simulink model "LQSwingup"  (R2019b)
settings: Solver=ode1  StartTime=0.0  StopTime=inf  FixedStep=0.002  RelTol=1e-3  EnableMultiTasking=on
PostLoadFcn:
  | qc_set_target_type(getConfigSet(bdroot, 'QUARC Default Target Configuration'));
undefined symbols (not defined in the file): HIL, Klqi_int, Klqi_state, Parameters, qc_get_step_size
libraries: quarc_library x4
settings Model: SimulationMode=external  ExtModeTrigDuration=5000  Creator=CFulford  LastModifiedBy=Student
settings SolverCC: PositivePriorityOrder=on
settings DataIOCC: LimitDataPoints=on  SaveFormat=Array  SignalLoggingSaveFormat=ModelDataLogs  ReturnWorkspaceOutputs=off
settings OptimizationCC: ExpressionDepthLimit=2147483647  InitFltsAndDblsToZero=on  LifeSpan=inf
settings DebuggingCC: SaveWithParameterizedLinksMsg=none  UnderspecifiedInitializationDetection=Classic  MergeDetectMultiDrivingBlocksExec=none  SolverPrmCheckMsg=warning  MultiTaskDSMMsg=warning  MultiTaskCondExecSysMsg=none  FcnCallInpInsideContextMsg=warning  StateNameClashWarn=warning  SFUnexpectedBacktrackingDiag=warning  SFNoUnconditionalDefaultTransitionDiag=warning  SFExecutionAtInitializationDiag=none  ArithmeticOperatorsInVariantConditions=warning
settings HardwareCC: ProdBitPerPointer=32  ProdBitPerSizeT=32  ProdBitPerPtrDiffT=32  ProdLargestAtomicFloat=None  ProdIntDivRoundTo=Undefined  ProdEndianess=Unspecified  ProdWordSize=32  ProdHWDeviceType=32-bit Generic
settings ModelReferenceCC: PropagateSignalLabelsOutOfModel=off
settings SFSimCC: SimUseLocalCustomCode=off  CustomCodeUndefinedFunction=UseInterfaceOnly
settings RTWCC: Description=QUARC Win64 Target  SystemTargetFile=quarc_win64.tlc  TemplateMakefile=quarc_default_tmf  RTWUseLocalCustomCode=off
settings CodeAppCC: StateflowObjectComments=on
settings STFCustomTargetCC: TargetPreCompLibLocation=C:\PROGRA~3\QUARC\lib\2019b\win64\release  ConcurrentExecutionCompliant=on  GeneratePreprocessorConditionals=Disable all  CombineOutputUpdateFcns=on  CPPClassGenCompliant=on  SystemTargetFile=quarc_win64.tlc
settings GRTTargetCC: TargetPreCompLibLocation=C:\PROGRA~3\QUARC\lib\2019b\win64\release  TargetLangStandard=C89/C90 (ANSI)  ParMdlRefBuildCompliant=off  CompOptLevelCompliant=off  GeneratePreprocessorConditionals=Disable all  MatFileLogging=off  UseToolchainInfoCompliant=off  ExtMode=on  ExtModeMexFile=quarc_comm
settings ConfigComp: CovMetricSettings=dw  CovHtmlReporting=on  CovSaveCumulativeToWorkspaceVar=on  CovSaveSingleToWorkspaceVar=on  CovExternalEMLEnable=off  CovSFcnEnable=off

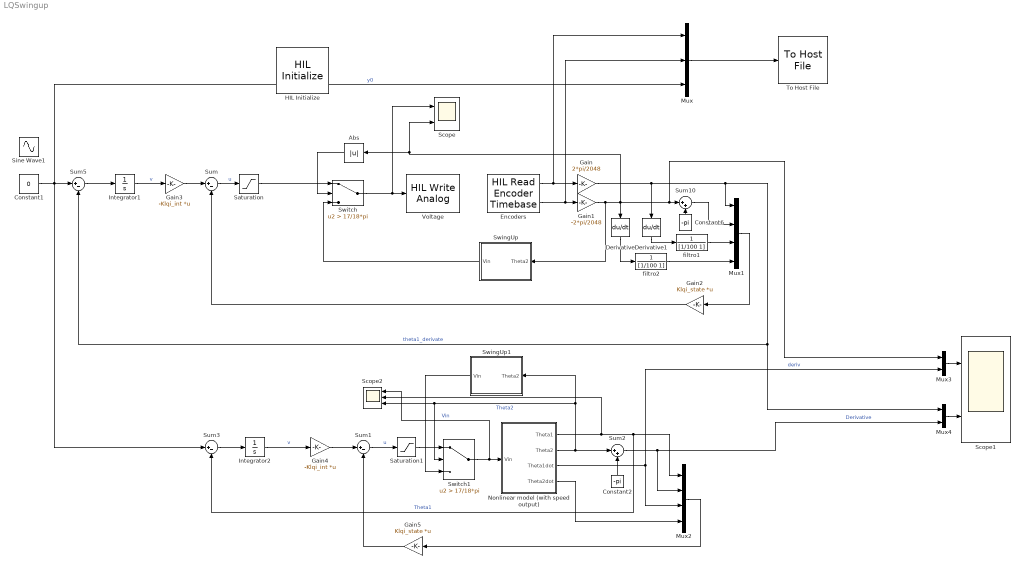
== system LQSwingup ==
  Abs : Abs
  Constant1 : Constant  Value=0
  Constant2 : Constant  Value=-pi
  Constant6 : Constant  Value=-pi
  Derivative : Derivative
  Derivative1 : Derivative
  Encoders : quarc_library/Data Acquisition/Generic/Timebases/HIL Read Encoder Timebase  object_name=HIL-1  clock=0  channels=[0:1]  samples_in_buffer=max(ceil(1/qc_get_step_size), 1)  active=on  vector_output=off  data_type_mode=Inherit via back propagation  data_type=double
  Gain : Gain  Gain=2*pi/2048
  Gain1 : Gain  Gain=-2*pi/2048
  Gain2 : Gain  Gain=Klqi_state  Multiplication=Matrix(K*u)
  Gain3 : Gain  Gain=-Klqi_int  Multiplication=Matrix(K*u)
  Gain4 : Gain  Gain=-Klqi_int  Multiplication=Matrix(K*u)
  Gain5 : Gain  Gain=Klqi_state  Multiplication=Matrix(K*u)
  HIL Initialize : quarc_library/Data Acquisition/Generic/Configuration/HIL Initialize  Priority=-99  object_name=HIL-1  board_type=qube_servo2_usb  board_number=0  board_options=""  exclusive=off  active=off  hardware_clocks=[0]  clock_modes=[]  initial_clock_frequencies=[]  set_clock_params_at_start=off  set_clock_params_at_switch_in=off  set_clock_frequencies_at_start=off  set_clock_frequencies_at_switch_in=off  analog_input_channels=[0]  analog_input_configurations=[]  analog_input_maximums=3  analog_input_minimums=-3  set_analog_input_params_at_start=off  set_analog_input_params_at_switch_in=off  analog_output_channels=[0]  analog_output_maximums=15  analog_output_minimums=-15  initial_analog_outputs=[0]  final_analog_outputs=[0]  watchdog_analog_outputs=0  set_analog_output_params_at_start=off  set_analog_output_params_at_switch_in=off  set_analog_outputs_at_start=on  set_analog_outputs_at_switch_in=off  set_analog_outputs_at_terminate=on  set_analog_outputs_at_switch_out=off  set_analog_outputs_on_watchdog=on  digital_input_channels=[]  digital_output_channels=[0]  digital_output_configuration=[]  initial_digital_outputs=[1]  final_digital_outputs=[0]  watchdog_digital_outputs=[0]  set_digital_output_params_at_start=off  set_digital_output_params_at_switch_in=off  set_digital_outputs_at_start=on  set_digital_outputs_at_switch_in=off  set_digital_outputs_at_terminate=on  set_digital_outputs_at_switch_out=off  set_digital_outputs_on_watchdog=on  encoder_channels=[0:1]  quadrature=[4]  encoder_filter_frequency=[]  initial_encoder_counts=[0]  set_encoder_params_at_start=off  set_encoder_params_at_switch_in=off  set_encoder_counts_at_start=on  set_encoder_counts_at_switch_in=off  pwm_channels=[]  pwm_modes=[]  pwm_frequency=[]  pwm_configuration=[]  pwm_alignment=[]  pwm_polarity=[]  pwm_leading_deadband=[]  pwm_trailing_deadband=[]  initial_pwm_outputs=[]  final_pwm_outputs=[]  watchdog_pwm_outputs=[]  set_pwm_params_at_start=off  set_pwm_params_at_switch_in=off  set_pwm_outputs_at_start=off  set_pwm_outputs_at_switch_in=off  set_pwm_outputs_at_terminate=off  set_pwm_outputs_at_switch_out=off  set_pwm_outputs_on_watchdog=off  other_output_channels=[11000:11002]  initial_other_outputs=[0 1 0]  final_other_outputs=[1 0 0]  watchdog_other_outputs=[0 0 1]  set_other_outputs_at_start=on  set_other_outputs_at_switch_in=off  set_other_outputs_at_terminate=on  set_other_outputs_at_switch_out=off  set_other_outputs_on_watchdog=on
  Integrator1 : Integrator
  Integrator2 : Integrator
  Mux : Mux  Inputs=3
  Mux1 : Mux
  Mux2 : Mux
  Mux3 : Mux  Inputs=2
  Mux4 : Mux  Inputs=2
  Nonlinear model (with speed output) : Subsystem
  Saturation : Saturate  UpperLimit=10  LowerLimit=-10
  Saturation1 : Saturate  UpperLimit=10  LowerLimit=-10
  Scope : Scope  NumInputPorts=2
  Scope1 : Scope  NumInputPorts=2
  Scope2 : Scope  NumInputPorts=3
  Sine Wave1 : Sin  SampleTime=0
  Sum{,1,3,5} (4 alike) : Sum  Inputs=|+-
  Sum10 : Sum  Inputs=|++
  Sum2 : Sum  Inputs=|++
  SwingUp : Subsystem
  SwingUp1 : Subsystem
  Switch : Switch  Criteria=u2 > Threshold  Threshold=17/18*pi
  Switch1 : Switch  Criteria=u2 > Threshold  Threshold=17/18*pi
  To Host File : quarc_library/Sinks/To Host/To Host File  file_name=data_%{date}_%{time}.mat  variable_name=data_%{date}_%{time}  decimation=1  sample_time=-1  file_format=MAT-file v.5  options=No header or footer  append=off  final_file_name=data_17-May-2024_12-50-43.mat  bitrate=2000000
  Voltage : quarc_library/Data Acquisition/Generic/Immediate I//O/HIL Write Analog  object_name=HIL-1  channels=0  sample_time=-1  active=off  vector_input=off
  "filtro1 " : TransferFcn  Denominator=[1/100 1]
  filtro2 : TransferFcn  Denominator=[1/100 1]
  wires:
  Mux/1 -> To Host File/1
  Gain2/1 -> Sum/2
  Encoders/2 -> Mux/2, Gain1/1
  Switch/1 -> Scope/1, Voltage/1
  Mux1/1 -> Gain2/1
  Mux3/1 -> Scope1/1
  "filtro1 "/1 -> Mux1/3
  Sum10/1 -> Mux1/2
  Gain3/1 -> Sum/1
  Derivative/1 -> filtro2/1
  Mux4/1 -> Scope1/2
  Derivative1/1 -> "filtro1 "/1
  Encoders/1 -> Mux/1, Gain/1
  Sum/1 -> Saturation/1  "u"
  Integrator1/1 -> Gain3/1  "v"
  filtro2/1 -> Mux1/4
  Gain/1 -> Sum5/2, Mux4/1, Mux1/1, Derivative1/1  "theta1_derivate"
  Sum5/1 -> Integrator1/1
  Constant6/1 -> Sum10/2
  Saturation/1 -> Switch/1
  Gain1/1 -> SwingUp/1(Theta2), Scope/2, Abs/1, Mux3/1, Sum10/1, Derivative/1
  SwingUp/1(Vin) -> Switch/3
  Nonlinear model (with speed output)/1(Theta1) -> Scope2/2, Mux2/1, Sum3/2  "Theta1"
  Saturation1/1 -> Switch1/1
  SwingUp1/1(Vin) -> Switch1/3
  Sum1/1 -> Saturation1/1  "u"
  Switch1/1 -> Scope2/1, Nonlinear model (with speed output)/1(Vin)  "Vin"
  Constant1/1 -> Mux/3, Sum3/1, Sum5/1  "y0"
  Nonlinear model (with speed output)/2(Theta2) -> Sum2/1, SwingUp1/1(Theta2), Switch1/2, Scope2/3  "Theta2"
  Nonlinear model (with speed output)/4(Theta2dot) -> Mux2/4
  Constant2/1 -> Sum2/2
  Nonlinear model (with speed output)/3(Theta1dot) -> Mux3/2, Mux2/3  "deriv"
  Sum3/1 -> Integrator2/1
  Sum2/1 -> Mux4/2, Mux2/2  "Derivative"
  Gain5/1 -> Sum1/2
  Integrator2/1 -> Gain4/1  "v"
  Mux2/1 -> Gain5/1
  Gain4/1 -> Sum1/1
  Abs/1 -> Switch/2

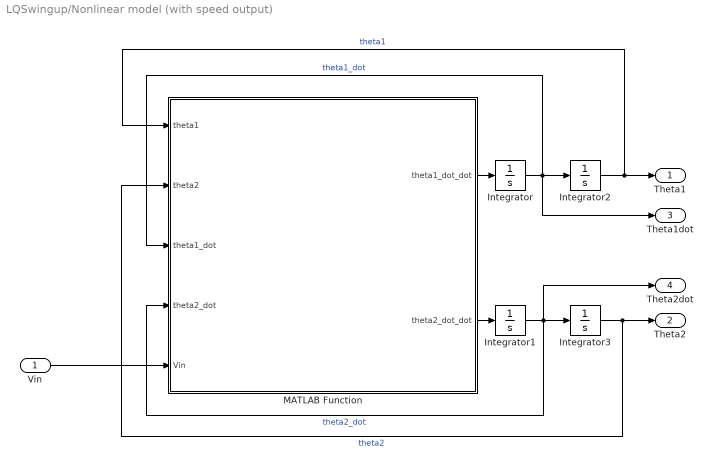
== system LQSwingup/Nonlinear model (with speed output) ==
  Vin : Inport
  Integrator{,1..3} (4 alike) : Integrator
  MATLAB Function : MATLAB Function  TreatAsAtomicUnit=on  mask{Pars=Parameters}
      mask prompts: Pars "Struct containing model parameters"
  Theta1 : Outport
  Theta2 : Outport  Port=2
  Theta1dot : Outport  Port=3
  Theta2dot : Outport  Port=4
  wires:
  Integrator/1 -> Theta1dot/1, MATLAB Function/3(theta1_dot), Integrator2/1  "theta1_dot"
  Integrator1/1 -> Theta2dot/1, MATLAB Function/4(theta2_dot), Integrator3/1  "theta2_dot"
  MATLAB Function/1(theta1_dot_dot) -> Integrator/1
  Integrator3/1 -> Theta2/1, MATLAB Function/2(theta2)  "theta2"
  MATLAB Function/2(theta2_dot_dot) -> Integrator1/1
  Integrator2/1 -> MATLAB Function/1(theta1), Theta1/1  "theta1"
  Vin/1 -> MATLAB Function/5(Vin)

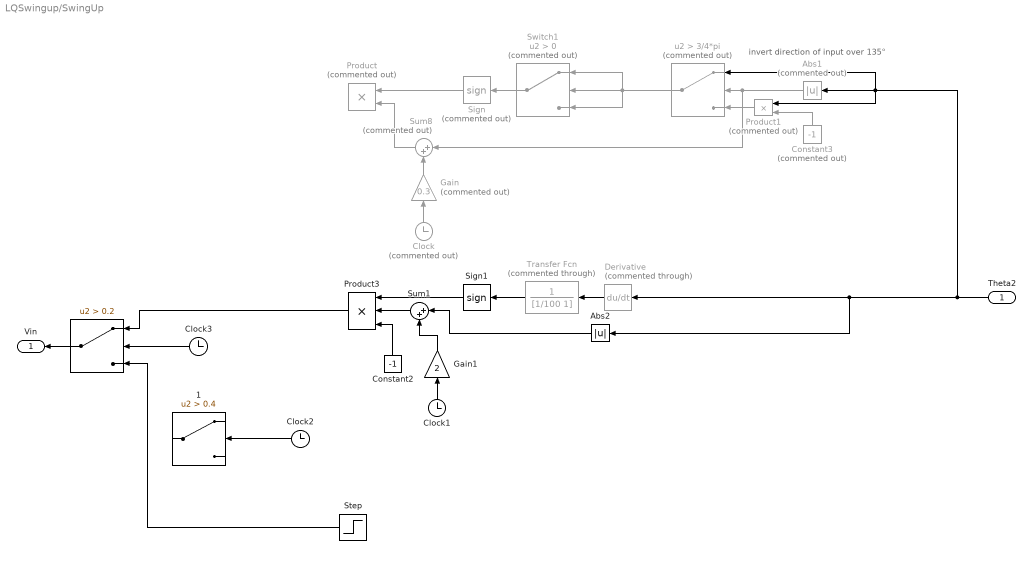
== system LQSwingup/SwingUp ==
  note: invert direction of input over 135°
  Theta2 : Inport
  " " : Switch  Commented=on  Criteria=u2 > Threshold  Threshold=3/4*pi
  " " : Switch  Criteria=u2 > Threshold  Threshold=0.2
  " 1" : Switch  Criteria=u2 > Threshold  Threshold=0.4
  Abs1 : Abs  Commented=on
  Abs2 : Abs
  Clock : Clock  Commented=on
  Clock1 : Clock
  Clock2 : Clock
  Clock3 : Clock
  Constant2 : Constant  Value=-1
  Constant3 : Constant  Commented=on  Value=-1
  Derivative : Derivative  Commented=through
  Gain : Gain  Commented=on  Gain=0.3
  Gain1 : Gain  Gain=2
  Product : Product  Commented=on
  Product1 : Product  Commented=on
  Product3 : Product  Inputs=3
  Sign : Signum  Commented=on
  Sign1 : Signum
  Step : Step  Time=0  SampleTime=0
  Sum1 : Sum  Inputs=|++
  Sum8 : Sum  Commented=on  Inputs=|++
  Switch1 : Switch  Commented=on  Criteria=u2 > Threshold
  Transfer Fcn : TransferFcn  Commented=through  Denominator=[1/100 1]
  Vin : Outport
  wires:
  Abs1/1 -> Sum8/1, " "/2
  " "/1 -> Switch1/3, Switch1/2, Switch1/1
  Constant3/1 -> Product1/2
  Clock/1 -> Gain/1
  Product1/1 -> " "/3
  Switch1/1 -> Sign/1
  Gain/1 -> Sum8/2
  Sign/1 -> Product/1
  Sum8/1 -> Product/2
  Sign1/1 -> Product3/1
  Sum1/1 -> Product3/2
  Clock1/1 -> Gain1/1
  Gain1/1 -> Sum1/2
  Constant2/1 -> Product3/3
  " "/1 -> Vin/1
  Product3/1 -> " "/1
  Clock2/1 -> " 1"/2
  Clock3/1 -> " "/2
  Abs2/1 -> Sum1/1
  Theta2/1 -> Product1/1, Abs1/1, " "/1, Derivative/1, Abs2/1
  Derivative/1 -> Transfer Fcn/1
  Transfer Fcn/1 -> Sign1/1
  Step/1 -> " "/3

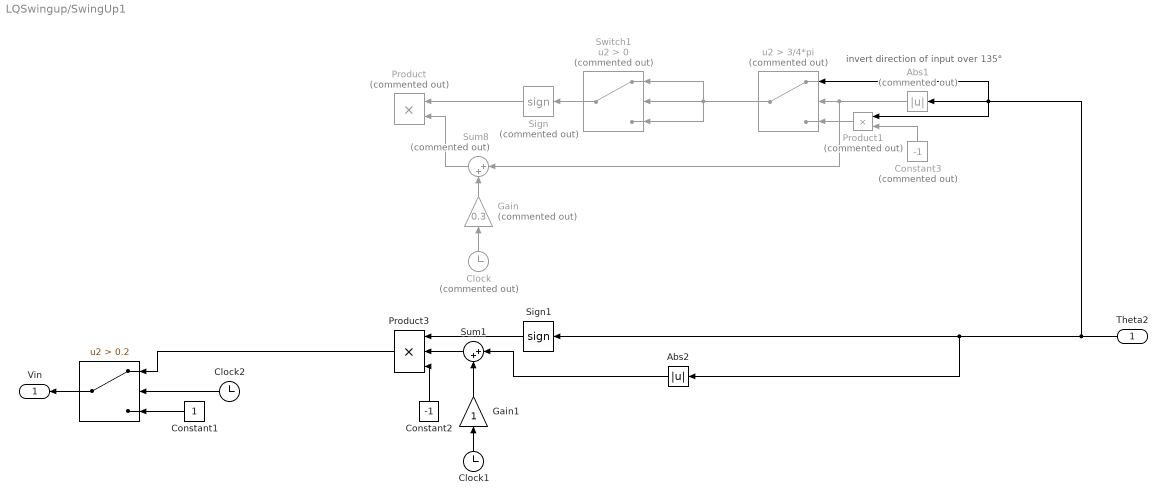
== system LQSwingup/SwingUp1 ==
  note: invert direction of input over 135°
  Theta2 : Inport
  " " : Switch  Commented=on  Criteria=u2 > Threshold  Threshold=3/4*pi
  " " : Switch  Criteria=u2 > Threshold  Threshold=0.2
  Abs1 : Abs  Commented=on
  Abs2 : Abs
  Clock : Clock  Commented=on
  Clock1 : Clock
  Clock2 : Clock
  Constant1 : Constant
  Constant2 : Constant  Value=-1
  Constant3 : Constant  Commented=on  Value=-1
  Gain : Gain  Commented=on  Gain=0.3
  Gain1 : Gain
  Product : Product  Commented=on
  Product1 : Product  Commented=on
  Product3 : Product  Inputs=3
  Sign : Signum  Commented=on
  Sign1 : Signum
  Sum1 : Sum  Inputs=|++
  Sum8 : Sum  Commented=on  Inputs=|++
  Switch1 : Switch  Commented=on  Criteria=u2 > Threshold
  Vin : Outport
  wires:
  Abs1/1 -> Sum8/1, " "/2
  " "/1 -> Switch1/3, Switch1/2, Switch1/1
  Constant3/1 -> Product1/2
  Clock/1 -> Gain/1
  Product1/1 -> " "/3
  Switch1/1 -> Sign/1
  Gain/1 -> Sum8/2
  Sign/1 -> Product/1
  Sum8/1 -> Product/2
  Sign1/1 -> Product3/1
  Sum1/1 -> Product3/2
  Clock1/1 -> Gain1/1
  Gain1/1 -> Sum1/2
  Theta2/1 -> Product1/1, Abs1/1, " "/1, Abs2/1, Sign1/1
  Abs2/1 -> Sum1/1
  Constant2/1 -> Product3/3
  Clock2/1 -> " "/2
  Constant1/1 -> " "/3
  " "/1 -> Vin/1
  Product3/1 -> " "/1

== matlab function LQSwingup/Nonlinear model (with speed output)/MATLAB Function ==
  data: theta1 input; theta1_dot_dot output; theta2 input; theta1_dot input; theta2_dot input; Vin input; theta2_dot_dot output; Pars parameter
function [theta1_dot_dot,theta2_dot_dot] = fcn(theta1, theta2, theta1_dot, theta2_dot,Vin, Pars)

   k1 = Pars.Jeq + Pars.m2*(Pars.l1^2 + Pars.x2^2*sin(theta2)^2);
   k2 = Pars.m2*Pars.l1*Pars.x2*cos(theta2);
   k3 = 2*Pars.m2*Pars.x2^2*sin(theta2)*cos(theta2)*theta1_dot*theta2_dot - Pars.m2*Pars.l1*Pars.x2*sin(theta2)*theta2_dot^2 +Pars.Ks*theta1 - Pars.Km/Pars.Rm*Vin + (Pars.Km^2)/Pars.Rm*theta1_dot + Pars.Kf1*theta1_dot;
   k4 = Pars.m2*Pars.l1*Pars.x2*cos(theta2);
   k5 = Pars.m2*Pars.x2^2 + Pars.I2;
   k6 = - Pars.m2*Pars.x2^2*sin(theta2)*cos(theta2)*theta1_dot^2 + Pars.m2*Pars.g*Pars.x2*sin(theta2) + Pars.Kf2*theta2_dot;


theta1_dot_dot = (k2*k6 - k3*k5)/(k1*k5 - k2*k4);
theta2_dot_dot = -(k1*k6 - k3*k4)/(k1*k5 - k2*k4);
